simulink model "VFlexP"  (R2024a)
settings: Solver=ode23tb  StartTime=0.0  StopTime=3  FixedStep=1e-5
model workspace (MAT data in the model file):
  DCop_DCBUCK : object (value not decoded)
  Grid_CCVSC_idx = [2; 3; 4; 5; 6; 7; 8; 9; 10; 11; 12]
  Grid_CCVSCs = 1
  Grid_CCVSCs_buses = 1
  Grid_CCVSCs_toM = [0 1 0 0 0 0 0 0 0 0 0 0 ... (781 elements, 71x11)]
  Grid_C_Lines = [0 0]
  Grid_Cbuses = [0.00666666666667 0.00666666666667 0.00666666666667]
  Grid_DC : object (value not decoded)
  Grid_DCop_DCBUCK : object (value not decoded)
  Grid_DCop_DC_PES : object (value not decoded)
  Grid_DFIGs = 1
  Grid_DFIGs_buses = 1
  Grid_DGs : string (value not decoded)
  Grid_From_buses = [1 2]
  Grid_GFls = 1
  Grid_GFls_buses = 1
  Grid_GFr_idx = 1
  Grid_GFrs = 1
  Grid_GFrs_buses = 1
  Grid_GFrs_toM = [1; 0; 0]
  Grid_IG_idx = 2
  Grid_IGs = 1
  Grid_IGs_buses = 1
  Grid_IGs_toM = [0; 1]
  Grid_L_Lines = [0.05 0.05]
  Grid_L_Loads = 0
  Grid_Lines_fromM : object (value not decoded)
  Grid_Lines_toM : object (value not decoded)
  Grid_Load_buses = []
  Grid_Load_busesDC = []
  Grid_MSGs = 1
  Grid_MSGs_buses = 1
  Grid_Nbuses = 3
  Grid_PQ_gen = 3
  Grid_Ploads = []
  Grid_PloadsDC = []
  Grid_Ps_lf = -0.138475313333
  Grid_Qloads = []
  Grid_Qs_lf = 0.00594619333333
  Grid_R_Lines = [0.005 0.005]
  Grid_R_Loads = 0
  Grid_R_Loads_DC = 0
  Grid_Rcf = [150 150 150]
  Grid_SCs = 1
  Grid_SCs_buses = 1
  Grid_SG_idx = 1
  Grid_SGs = 1
  Grid_SGs_buses = 1
  Grid_SGs_toM = [1; 0]
  Grid_To_buses = [2 3]
  Grid_VCVSC_idx = [1; 2; 3; 4; 5; 6; 7; 8; 9; 10; 11; 12]
  Grid_VCVSCs = 1
  Grid_VCVSCs_buses = [1; 2; 3; 6; 8; 9; 12; 58; 59; 60; 63; 65]
  Grid_VCVSCs_toM = [1 0 0 0 0 0 0 0 0 0 0 0 ... (852 elements, 71x12)]
  Grid_VSM_idx = 2
  Grid_VSMs = 1
  Grid_VSMs_buses = 1
  Grid_VSMs_toM = [0; 1]
  Grid_admitt_matrix = [1.9801990198-19.801979198i  -1.9801980198+19.801980198i; -1.9801980198+19.801980198i  1.9801990198-19.801979198i]
  Grid_admitt_matrix_noloads = [1.9801990198-19.801979198i  -1.9801980198+19.801980198i; -1.9801980198+19.801980198i  1.9801990198-19.801979198i]
  Grid_bus = [1; 2; 3]
  Grid_busDC_complexity = 1
  Grid_busDC_complexity_PF = 2
  Grid_bus_complexity = [1 1 1]
  Grid_bus_complexity_PF = [1 1 1]
  Grid_buses_lf = 1
  Grid_conductance_matrix = 0.00666666666667
  Grid_conductance_matrix_noloads = 0.00666666666667
  Grid_fref : object (value not decoded)
  Grid_gen_static_params : mBase (value not decoded)
  Grid_iPs_lf = -7.22150378958
  Grid_iQs_lf = 168.17482109
  Grid_iadmitt_matrix = [250000.001075-249999.987531i  249999.998575-250000.012531i; 249999.998575-250000.012531i  250000.001075-249999.987531i]
  Grid_iadmitt_matrix_noloads = [250000.001075-249999.987531i  249999.998575-250000.012531i; 249999.998575-250000.012531i  250000.001075-249999.987531i]
  Grid_iconductance_matrix = 150
  Grid_iconductance_matrix_noloads = 150
  Grid_init_OK_bool = 1
  Grid_intconv_PF : object (value not decoded)
  Grid_lf_op : op_report (value not decoded)
  Grid_lineDC_complexity = []
  Grid_lineDC_complexity_PF = []
  Grid_line_complexity = [1 1]
  Grid_line_complexity_PF = [3 3]
  Grid_loadDC_complexity = []
  Grid_loadDC_complexity_PF = []
  Grid_load_complexity = []
  Grid_load_complexity_PF = []
  Grid_opDC_CCVSC : object (value not decoded)
  Grid_opDC_VSM : object (value not decoded)
  Grid_opGFr : object (value not decoded)
  Grid_opVCVSC : object (value not decoded)
  Grid_op_CCVSC : object (value not decoded)
  Grid_op_IG : object (value not decoded)
  Grid_op_SG : object (value not decoded)
  Grid_op_VSM : object (value not decoded)
  Grid_shift_lines = [0 0]
  Grid_tap_lines = [1 1]
  Grid_v_buses_mod = [1 1.0001218564 1]
  LinsysParamChangeStruct : Param1 (value not decoded)
  Lline = 0.01
  Rline = 1e-05
  linsys : object (value not decoded)
symbols that are objects in the model workspace (value not decoded): Grid_DCop_DC_PES, Grid_DCop_DCBUCK, Grid_op_CCVSC, Grid_op_IG, Grid_op_SG, Grid_op_VSM, Grid_opDC_CCVSC, Grid_opDC_VSM, Grid_opGFr, Grid_opVCVSC
undefined symbols (not defined in the file or in its folder): block_buses_DC, block_idx, CCVSC_idx, Cf, costs, costs2, DFIGs_nodes, DiscIntNeverNeededParam, entity, Fb, Fi, From_nodes, Grid_op_DFIG, Grid_op_DFIG_PQ, Grid_op_MSG, Grid_op_SC, Grid_op_VCVSC, Kic, Kiv, Kpc, Kpv, last_send, Lc, Lf, m, Matrix_flux_to_i, mD, mp, MSGs_buses, Nbuses_DC, nq, op_VCVSC, Psche, Rc, Rf, rkq1, rkq2, SCs_buses, SCs_nodes, sec_control_structure, set_DG_up, set_extra_satur, set_sending_cost, SGs_buses, SGs_nodes, Tf, To_nodes, VI_L, VI_R, WOF_Tf, xkq1, xkq2
libraries: simulink x447, eeGeneralControl x5
(part 2 of 30)

== system VFlexP/Grid/Dynamic/DCAC converters ==
  note: mdlWks = get_param(bdroot,'ModelWorkspace'); % Get the model workspace
      | block_name = get_param(gcb,'Name');
      | bvarname = get_param(get_param(get_param(get_param(...
      | gcb, 'Parent'), 'Parent'), 'Parent'), 'bvarname');
      | DC = mdlWks.getVariable([bvarname 'DC']);
      | try
      | block_DC_buses = DC.(block_name + "s_DC_buses");
      | block_buses = DC.(block_name + "s_buses");
      | block_DC_toM = DC.(block_name + "s_DC_toM");
      | block_toM = DC.(block_name + "s_toM");
      | dparams = DC.(block_name + "_dparams");
      | fref = mdlWks.getVariable([bvarname 'fref']);
      | block_fref = fref.(block_name);
      | catch ME
      | errordlg(ME.message)
      | end
  vac : Inport
  vdc : Inport  Port=2
  DC_CCVSC : Subsystem  Commented=on  mask(CCVSC){Pmax=0, Qmax=0, fb=50, dynamic_CC=Dynamic, Tint=0.1, Kint=1, Bint=1, dynamic_PLL=Dynamic, kpi=1, kii=10, Tf=0.01, alphapcoef=0, alphaqcoef=0, Prel=1, Qrel=1, Eref=1, kp=10, kq=10}
      mask prompts: Pmax "Active power limit (p.u.)"; Qmax "Reactive power limit (p.u.)"; fb "Base frequency (Hz)"; dynamic_CC "Dynamic behaviour"; dynamic_PLL "Dynamic behaviour"; Tf "LPF time constant (s)"; alphapcoef "P droop coefficient"; alphaqcoef "Q droop coefficient"; Prel "P/P_NmP"; Qrel "Q/Q_NnQ"; Eref "Nominal voltage of PCC"; kp "P gain"; kq "Q gain"
      mask help: Grid-following converter. CC is the current controller. Dynamic behavior includes the PI controller, decoupling and output inductance. Static behavior consists of setting the reference current directly in the output. PC is the power controller including the current reference calculation and low-pass filters for the power measurements.
      mask init:
      | mdlWks = get_param(bdroot,'ModelWorkspace'); % Get the model workspace
      | block_name = get_param(gcb,'Name');
      | bvarname = get_param(get_param(get_param(get_param(...
      |         gcb, 'Parent'), 'Parent'), 'Parent'), 'bvarname');
      | DC = mdlWks.getVariable([bvarname 'DC']);
      | try
      |     block_DC_buses = DC.(block_name + "s_DC_buses");
      |     block_buses = DC.(block_name + "s_buses");
      |     block_DC_toM = DC.(block_name + "s_DC_toM");
      |     block_toM = DC.(block_name + "s_toM");
      |     dparams = DC.(block_name + "_dparams");
      |     fref = mdlWks.getVariable([bvarname 'fref']);
      |     block_fref = fref.(block_name);
      | catch ME
      |     %errordlg(ME.message) 
      | end
      | 
      | 
      | block = gcb;
      | if Tf ~= 0
      |     iTf = 1/Tf;
      |     set_param([block '/PC/LPF_d'],'Commented','off')
      |     set_param([block '/PC/LPF_q'],'Commented','off')
      |     set_param([block '/LPF_d'],'Commented','off')
      |     set_param([block '/LPF_q'],'Commented','off')
      | else
      |     set_param([block '/PC/LPF_d'],'Commented','through')
      |     set_param([block '/PC/LPF_q'],'Commented','through')
      |     set_param([block '/LPF_d'],'Commented','through')
      |     set_param([block '/LPF_q'],'Commented','through')
      | end
      mask Help: web('Documentation/CCVSC.html')
      mask TypeOptions dynamic_CC: Dynamic | Static
      mask Callback dynamic_CC:
      | block = gcb;
      | dynamic = get_param(block, 'dynamic_CC');
      | param_vis = get_param(block,'MaskVisibilities');
      | block_params = string(fieldnames(get_param(block, 'DialogParameters')));
      | switch dynamic
      |     case 'Dynamic'
      |         set_param([gcb '/CC'], 'LabelModeActiveChoice', 'dynamic')
      |         param_vis(find(block_params == 'Tint'):find(block_params == 'Rf')) = cellstr("on");
      |     case 'Static'
      |         set_param([gcb '/CC'], 'LabelModeActiveChoice', 'static')
      |         param_vis(find(block_params == 'Tint'):find(block_params == 'Rf')) = cellstr("off");
      | end
      | set_param(block,'MaskVisibilities',param_vis)
      mask TypeOptions dynamic_PLL: Dynamic | Static
      mask Callback dynamic_PLL:
      | block = gcb;
      | dynamic = get_param(block, 'dynamic_PLL');
      | param_vis = get_param(block,'MaskVisibilities');
      | block_params = string(fieldnames(get_param(block, 'DialogParameters')));
      | switch dynamic
      |     case 'Dynamic'
      |         set_param([gcb '/PLL'], 'LabelModeActiveChoice', 'dynamic')
      |         param_vis(find(block_params == 'kpi'):find(block_params == 'kii')) = cellstr("on");
      |     case 'Static'
      |         set_param([gcb '/PLL'], 'LabelModeActiveChoice', 'static')
      |         param_vis(find(block_params == 'kpi'):find(block_params == 'kii')) = cellstr("off");
      | end
      | set_param(block,'MaskVisibilities',param_vis)
      mask DialogControl CC Prompt: CC
      mask DialogControl PLL Prompt: PLL
      mask DialogControl PC Prompt: PC
      mask DialogControl SC Prompt: SC
  DC_VCVSC : Subsystem  Commented=on  mask(VCVSC){Pmax=Inf, Qmax=Inf, fb=50, dynamic_VCC=Static, Lf=0.01, Rf=0.001, Rcf=1000000, Cfi=0.1, Kint=1, Tint=0.1, Bint=1, Kext=1, Bext=1, Text=0.1, Fi=1, Tf=0.01, mp=0.01, nq=0.01, VI_L=0.1, VI_R=0.01, WOF_Tf=0, cf=0.1, cv=0.1, L_out=0.1, R_out=0.01}
      mask prompts: Pmax "Active power limit (p.u.)"; Qmax "Reactive power limit (p.u.)"; fb "Base frequency (Hz)"; dynamic_VCC "Dynamic behavior"; Lf "Filter inductance (pu)"; Rf "Filter resistance (pu)"; Rcf "Parallel resistance to C (pu)"; Cfi "Filter capacitance (pu)"; Fi "Current feedfordward gain"; Tf "Low-pass filter time constant (s)"; mp "Droop coefficient mp (pu)"; nq "Droop coefficient nq (pu)"; VI_L "Inductance (pu)"; VI_R "Resistance (pu)"; WOF_Tf "WOF time constant (s)"; cf "Frequency SC gain"; cv "Voltage SC gain"; L_out "Output inductance (p.u.)"; R_out "Output resistance (p.u.)"
      mask help: Grid-forming converter. VCC are the voltage and current controllers. Dynamic behavior includes the PI controllers, decoupling, current feedfordward and LC output filter. Static behavior consists of setting the reference voltage directly in the output. PC is the power controller including the droop control and low-pass filters for the power measurements.
      mask init:
      | mdlWks = get_param(bdroot,'ModelWorkspace'); % Get the model workspace
      | block_name = get_param(gcb,'Name');
      | bvarname = get_param(get_param(get_param(get_param(...
      |         gcb, 'Parent'), 'Parent'), 'Parent'), 'bvarname');
      | DC = mdlWks.getVariable([bvarname 'DC']);
      | try
      |     block_DC_buses = DC.(block_name + "s_DC_buses");
      |     block_buses = DC.(block_name + "s_buses");
      |     block_DC_toM = DC.(block_name + "s_DC_toM");
      |     block_toM = DC.(block_name + "s_toM");
      |     dparams = DC.(block_name + "_dparams");
      | catch ME
      |     %errordlg(ME.message)
      | end
      mask Help: web('Documentation/VCVSC.html')
      mask TypeOptions dynamic_VCC: Dynamic with limitation | Dynamic | Static | Dynamic VC and static CC
      mask Callback dynamic_VCC:
      | block = gcb;
      | dynamic = get_param(block, 'dynamic_VCC');
      | param_vis = get_param(block,'MaskVisibilities');
      | block_params = string(fieldnames(get_param(block, 'DialogParameters')));
      | switch dynamic
      |     case 'Dynamic'
      |         param_vis(find(block_params == 'Lf'):find(block_params == 'Fi')) = cellstr("on");
      |         set_param([gcb '/VCC'], 'LabelModeActiveChoice', 'dynamic');
      |     case 'Dynamic with limitation'
      |         param_vis(find(block_params == 'Lf'):find(block_params == 'Fi')) = cellstr("on");
      |         set_param([gcb '/VCC'], 'LabelModeActiveChoice', 'dynamic_limiting');
      |     case 'Static'
      |         param_vis(find(block_params == 'Lf'):find(block_params == 'Fi')) = cellstr("off");
      |         set_param([gcb '/VCC'], 'LabelModeActiveChoice', 'static');
      |     case 'Dynamic VC and static CC'
      |         param_vis(find(block_params == 'Lf'):find(block_params == 'Fi')) = cellstr("on");
      |         param_vis(ismember(block_params, ["Lf","Rf","Kpc","Kic","Fi"])) = cellstr("off");
      |         set_param([gcb '/VCC'], 'LabelModeActiveChoice', 'dynamic_VC');
      | end
      | set_param(block,'MaskVisibilities',param_vis)
      mask TypeOptions Tf: PC/Tf
      mask TypeOptions mp: PC/mp
      mask TypeOptions nq: PC/nq
      mask TypeOptions VI_L: VI/L
      mask TypeOptions VI_R: VI/R
      mask TypeOptions WOF_Tf: VI/Tf
      mask DialogControl Container8 Prompt: Parameters
      mask DialogControl VCC Prompt: VCC
      mask DialogControl PC Prompt: PC
      mask DialogControl VI Prompt: VI
      mask DialogControl SC Prompt: SC
      mask DialogControl Container9 Prompt: Others
  DC_VSM : Subsystem  mask(VCVSC){Hv=Tf/(2*mp), Dv=0, Pmax=Inf, Qmax=Inf, fb=50, dynamic_VCC=Static, Lf=Lf, Rf=Rf, Rcf=1000000, Cfi=Cf, Kint=Kpc, Tint=Kpc/Kic, Bint=1, Kext=Kpv, Bext=1, Text=Kpv/Kiv, Fi=Fi, Rv=mp, nq=0, VI_L=VI_L, VI_R=VI_R, WOF_Tf=WOF_Tf, cf=0.1, cv=0.1, L_out=Lc, R_out=Rc}
      mask prompts: Hv "Inertia"; Dv "Damping"; Pmax "Active power limit (p.u.)"; Qmax "Reactive power limit (p.u.)"; fb "Base frequency (Hz)"; dynamic_VCC "Dynamic behavior"; Lf "Filter inductance (pu)"; Rf "Filter resistance (pu)"; Rcf "Parallel resistance to C (pu)"; Cfi "Filter capacitance (pu)"; Fi "Current feedfordward gain"; Rv "Droop Rv"; nq "Droop nq"; VI_L "Inductance (pu)"; VI_R "Resistance (pu)"; WOF_Tf "WOF time constant (s)"; cf "Frequency SC gain"; cv "Voltage SC gain"; L_out "Output inductance (p.u.)"; R_out "Output resistance (p.u.)"
      mask help: Grid-forming converter. VCC are the voltage and current controllers. Dynamic behavior includes the PI controllers, decoupling, current feedfordward and LC output filter. Static behavior consists of setting the reference voltage directly in the output. PC is the power controller including the droop control and low-pass filters for the power measurements.
      mask init: same as VFlexP/Grid/Dynamic/DCAC converters/DC_VCVSC
      mask Help: web('Documentation/VCVSC.html')
      mask TypeOptions dynamic_VCC: Dynamic with limitation | Dynamic | Static | Dynamic VC and static CC
      mask Callback dynamic_VCC:
      | block = gcb;
      | dynamic = get_param(block, 'dynamic_VCC');
      | param_vis = get_param(block,'MaskVisibilities');
      | block_params = string(fieldnames(get_param(block, 'DialogParameters')));
      | switch dynamic
      |     case 'Dynamic'
      |         param_vis(find(block_params == 'Lf'):find(block_params == 'Fi')) = cellstr("on");
      |         set_param([gcb '/VCC'], 'LabelModeActiveChoice', 'dynamic');
      |     case 'Dynamic with limitation'
      |         param_vis(find(block_params == 'Lf'):find(block_params == 'Fi')) = cellstr("on");
      |         set_param([gcb '/VCC'], 'LabelModeActiveChoice', 'dynamic_limiting');
      |     case 'Static'
      |         param_vis(find(block_params == 'Lf'):find(block_params == 'Fi')) = cellstr("off");
      |         set_param([gcb '/VCC'], 'LabelModeActiveChoice', 'static');
      |     case 'Dynamic VC and static CC'
      |         param_vis(find(block_params == 'Lf'):find(block_params == 'Fi')) = cellstr("on");
      |         param_vis(ismember(block_params, ["Lf","Rf","Kpc","Kic","Fi"])) = cellstr("off");
      |         set_param([gcb '/VCC'], 'LabelModeActiveChoice', 'dynamic_VC');
      | end
      | set_param(block,'MaskVisibilities',param_vis)
      mask TypeOptions VI_L: VI/L
      mask TypeOptions VI_R: VI/R
      mask TypeOptions WOF_Tf: VI/Tf
      mask DialogControl Container8 Prompt: Parameters
      mask DialogControl VCC Prompt: VCC
      mask DialogControl PC Prompt: PC
      mask DialogControl VI Prompt: VI
      mask DialogControl SC Prompt: SC
      mask DialogControl Container9 Prompt: Others
  Sum : Sum  Inputs=|+++
  Sum1 : Sum  Inputs=|+++
  iac : Outport
  idc : Outport  Port=2
  wires:
  [vac] -> DC_CCVSC/1(vac)
  [vac] -> DC_VCVSC/1(vac)
  vac/1 -> [vac]
  DC_VCVSC/1(iac) -> Sum/1
  Sum/1 -> iac/1
  DC_CCVSC/1(iac) -> Sum/2
  [vdc] -> DC_VCVSC/2(vdc)
  DC_VCVSC/2(idc) -> Sum1/1
  Sum1/1 -> idc/1
  DC_CCVSC/2(idc) -> Sum1/2
  [vdc] -> DC_CCVSC/2(vdc)
  vdc/1 -> [vdc]
  [vdc] -> DC_VSM/2(vdc)
  [vac] -> DC_VSM/1(vac)
  DC_VSM/2(idc) -> Sum1/3
  DC_VSM/1(iac) -> Sum/3

== system VFlexP/Grid/Dynamic/Generators ==
  note: Include the following mask initialisation code for each unit:
  note: mdlWks = get_param(bdroot,'ModelWorkspace'); % Get the model workspace
      | block_name = get_param(gcb,'Name');
      | try
      | bvarname = get_param(get_param(get_param(get_param(...
      | gcb, 'Parent'), 'Parent'), 'Parent'), 'bvarname');
      | block_buses = mdlWks.getVariable([bvarname block_name 's_buses']);
      | block_idx = mdlWks.getVariable([bvarname block_name '_idx']);
      | block_toM = mdlWks.getVariable([bvarname block_name 's_toM']);
      | fref = mdlWks.getVariable([bvarname 'fref']);
      | block_fref = fref.(block_name);
      | catch ME % block in initialisation
      | %errordlg(ME.message)
      | try
      | block_buses = 1:length(mdlWks.getVariable([block_name 's_buses']));
      | block_idx = mdlWks.getVariable([block_name '_idx']);
      | block_toM = mdlWks.getVariable([block_name 's_toM']);
      | block_fref = 1;
      | catch ME
      | %errordlg(ME.message)
      | end
      | end
  v : Inport
  ref : Inport  Port=2
  DFIG : Subsystem  Commented=on  mask(Doubly Fed Induction Generator){DFIGs_nodes=DFIGs_nodes, FBASE=50, D=0, H=3.3, Ls_pu=0.1178, Rs_pu=0.00734, Lm_pu=4.709, Rr_pu=0.01225, Lr_pu=0.15349, Ra_pu=0.1, La_pu=1, Cf_pu=0.0555, Ki_ia=7162, Kp_ia=6.5, Ki_ir=2117, Kp_ir=1.96, Ki_vc2=-562.5, Kp_vc2=-5.25, Ki_s=12000, Kp_s=1200, Kp_pll=2.33, Ki_pll=877}
      mask prompts: FBASE "Base frequency (Hz)"; D "Damping (pu)"; H "Inertia (s)"; Ls_pu "Stator inductances (pu)"; Rs_pu "Stator resistances (pu)"; Lm_pu "Mutual inductance (pu)"; Rr_pu "Rotor Resistance (pu)"; Lr_pu "Rotor Inductance"; Ra_pu "Filter Resistance (pu)"; La_pu "Filter Inductance (pu)"; Cf_pu "DC-Link Capacitance"; Ki_ia "GSC Ki"; Kp_ia "GSC Kp"; Ki_ir "RSC Ki"; Kp_ir "RSC Kp"; Ki_vc2 "DC Link Voltage Control Ki"; Kp_vc2 "DC Link Voltage Control Kp"; Ki_s "Slip Control Ki"; Kp_s "Slip Control Kp"; Kp_pll "PLL Kp"; Ki_pll "PLL Ki"
      mask help: Doubly Fed Induction Generator modelled in d-q reference frame.
      mask init:
      | mdlWks = get_param(bdroot,'ModelWorkspace'); % Get the model workspace
      | block_name = get_param(gcb,'Name');
      | try
      |     bvarname = get_param(get_param(get_param(get_param(...
      |         gcb, 'Parent'), 'Parent'), 'Parent'), 'bvarname');
      |     block_buses = mdlWks.getVariable([bvarname block_name 's_buses']);
      | 	block_idx = mdlWks.getVariable([bvarname block_name '_idx']);
      | catch % block in initialisation
      |     try
      |         block_buses = 1:length(mdlWks.getVariable([block_name 's_buses']));
      | 	    block_idx = mdlWks.getVariable([block_name '_idx']);
      |     catch ME
      |         %errordlg(ME.message)
      |     end
      | end
      | 
      | 
      |     n = length(block_buses);
      |     Lbiginv = zeros(6*n,6*n); % La grande con las inversas en diagonal
      |     if length(Ls_pu) == 1
      |         Ls_pu = Ls_pu*ones(1, n);
      |     end
      |     if length(Lr_pu) == 1
      |         Lr_pu = Lr_pu*ones(1, n);
      |     end
      |     if length(Lm_pu) == 1
      |         Lm_pu = Lm_pu*ones(1, n);
      |     end
      |     if length(La_pu) == 1
      |         La_pu = La_pu*ones(1, n);
      |     end
      |     Lss_pu =  Ls_pu + Lm_pu;
      |     Lrr_pu = Lr_pu + Lm_pu;
      |     
      |     for i=1:n
      |         j = 6*(i-1)+1;
      |         L = [Lss_pu(i) 0 Lm_pu(i) 0 0 0;...
      |         0 Lss_pu(i) 0 Lm_pu(i) 0 0;...
      |         Lm_pu(i) 0 Lrr_pu(i) 0 0 0;...
      |         0 Lm_pu(i) 0 Lrr_pu(i) 0 0;...
      |         0 0 0 0 La_pu(i) 0;...
      |         0 0 0 0 0 La_pu(i)];
      |         Lbiginv(j:j+5, j:j+5) = inv(L);
      |     end
      | %     sigma = Lrr_pu-(Lm_pu^2)/Lss_pu;
      |     sigma =  1-Lm_pu.^2./(Lss_pu.*Lrr_pu);
      |     omega_base = FBASE*2*pi;
      mask Help: web([extractBefore(get_param(bdroot, 'filename'),gcs) 'Documentation/SM.html'])
      mask DialogControl Params Prompt: Parameters
      mask DialogControl Container10 Prompt: PI Parameters
      mask DialogControl Params_copy Prompt: Parameters
  GFl : Subsystem  Commented=on  mask(GFl){Pmax=0, Qmax=0, fb=50, dynamic_CC=Static, Tint=0.1, Kint=1, Bint=1, Lf=0.01, Rf=0.001, dynamic_PLL=Dynamic, kpi=1, kii=10, Tf=0, alphapcoef=0, alphaqcoef=0, Prel=1, Qrel=1, Eref=1}
      mask prompts: Pmax "Active power limit (p.u.)"; Qmax "Reactive power limit (p.u.)"; fb "Base frequency (Hz)"; dynamic_CC "Dynamic behaviour"; Lf "Filter inductance"; Rf "Filter resistance"; dynamic_PLL "Dynamic behaviour"; Tf "LPF time constant (s)"; alphapcoef "P droop coefficient"; alphaqcoef "Q droop coefficient"; Prel "P/P_NmP"; Qrel "Q/Q_NnQ"; Eref "Nominal voltage of PCC"
      mask help: Grid-following converter. CC is the current controller. Dynamic behavior includes the PI controller, decoupling and output inductance. Static behavior consists of setting the reference current directly in the output. PC is the power controller including the current reference calculation and low-pass filters for the power measurements.
      mask init:
      | mdlWks = get_param(bdroot,'ModelWorkspace'); % Get the model workspace
      | block_name = get_param(gcb,'Name');
      | try
      |     bvarname = get_param(get_param(get_param(get_param(...
      |         gcb, 'Parent'), 'Parent'), 'Parent'), 'bvarname');
      |     block_buses = mdlWks.getVariable([bvarname block_name 's_buses']);
      | 	block_idx = mdlWks.getVariable([bvarname block_name '_idx']);
      |     block_toM = mdlWks.getVariable([bvarname block_name 's_toM']);
      |     fref = mdlWks.getVariable([bvarname 'fref']);
      |     block_fref = fref.(block_name);
      | catch ME % block in initialisation
      |     %errordlg(ME.message)
      |     try
      |         block_buses = 1:length(mdlWks.getVariable([block_name 's_buses']));
      | 	    block_idx = mdlWks.getVariable([block_name '_idx']);
      |         block_toM = mdlWks.getVariable([block_name 's_toM']);
      |         block_fref = 1;
      |     catch ME
      |         %errordlg(ME.message)
      |     end
      | end
      | 
      | 
      | 
      | block = gcb;
      | if Tf ~= 0
      |     iTf = 1/Tf;
      |     set_param([block '/PC/LPF_d'],'Commented','off')
      |     set_param([block '/PC/LPF_q'],'Commented','off')
      |     set_param([block '/LPF_d'],'Commented','off')
      |     set_param([block '/LPF_q'],'Commented','off')
      | else
      |     set_param([block '/PC/LPF_d'],'Commented','through')
      |     set_param([block '/PC/LPF_q'],'Commented','through')
      |     set_param([block '/LPF_d'],'Commented','through')
      |     set_param([block '/LPF_q'],'Commented','through')
      | end
      mask Help: web('doc_GFl.html')
      mask TypeOptions dynamic_CC: Dynamic | Static
      mask Callback dynamic_CC:
      | block = gcb;
      | dynamic = get_param(block, 'dynamic_CC');
      | param_vis = get_param(block,'MaskVisibilities');
      | block_params = string(fieldnames(get_param(block, 'DialogParameters')));
      | switch dynamic
      |     case 'Dynamic'
      |         set_param([gcb '/CC'], 'LabelModeActiveChoice', 'dynamic')
      |         param_vis(find(block_params == 'Tint'):find(block_params == 'Rf')) = cellstr("on");
      |     case 'Static'
      |         set_param([gcb '/CC'], 'LabelModeActiveChoice', 'static')
      |         param_vis(find(block_params == 'Tint'):find(block_params == 'Rf')) = cellstr("off");
      | end
      | set_param(block,'MaskVisibilities',param_vis)
      mask TypeOptions dynamic_PLL: Dynamic | Static
      mask Callback dynamic_PLL:
      | block = gcb;
      | dynamic = get_param(block, 'dynamic_PLL');
      | param_vis = get_param(block,'MaskVisibilities');
      | block_params = string(fieldnames(get_param(block, 'DialogParameters')));
      | switch dynamic
      |     case 'Dynamic'
      |         set_param([gcb '/PLL'], 'LabelModeActiveChoice', 'dynamic')
      |         param_vis(find(block_params == 'kpi'):find(block_params == 'kii')) = cellstr("on");
      |     case 'Static'
      |         set_param([gcb '/PLL'], 'LabelModeActiveChoice', 'static')
      |         param_vis(find(block_params == 'kpi'):find(block_params == 'kii')) = cellstr("off");
      | end
      | set_param(block,'MaskVisibilities',param_vis)
      mask DialogControl CC Prompt: CC
      mask DialogControl PLL Prompt: PLL
      mask DialogControl PC Prompt: PC
  GFr : Subsystem  mask(GFr){Pmax=Inf, Qmax=Inf, fb=50, dynamic_VCC=Static, Lf=0.1, Rf=0.01, Rcf=1000000, Cfi=0.1, Kint=1, Tint=0.1, Bint=1, Kext=0.1, Bext=1, Text=0.1, Fi=1, Tf=Tf, mp=mp, mD=mD, nq=0.001, VI_L=0, VI_R=0, WOF_Tf=0, L_out=Lc, R_out=Rc}
      mask prompts: Pmax "Active power limit (p.u.)"; Qmax "Reactive power limit (p.u.)"; fb "Base frequency (Hz)"; dynamic_VCC "Dynamic behavior"; Lf "Filter inductance (pu)"; Rf "Filter resistance (pu)"; Rcf "Parallel resistance to C (pu)"; Cfi "Filter capacitance (pu)"; Fi "Current feedfordward gain"; Tf "Low-pass filter time constant (s)"; mp "Droop coefficient mp (pu)"; mD "Droop coefficient mD (pu)"; nq "Droop coefficient nq (pu)"; VI_L "Inductance (pu)"; VI_R "Resistance (pu)"; WOF_Tf "WOF time constant (s)"; L_out "Output inductance (p.u.)"; R_out "Output resistance (p.u.)"
      mask help: Grid-forming converter. VCC are the voltage and current controllers. Dynamic behavior includes the PI controllers, decoupling, current feedfordward and LC output filter. Static behavior consists of setting the reference voltage directly in the output. PC is the power controller including the droop control and low-pass filters for the power measurements.
      mask init:
      | mdlWks = get_param(bdroot,'ModelWorkspace'); % Get the model workspace
      | block_name = get_param(gcb,'Name');
      | try
      |     bvarname = get_param(get_param(get_param(get_param(...
      |         gcb, 'Parent'), 'Parent'), 'Parent'), 'bvarname');
      |     block_buses = mdlWks.getVariable([bvarname block_name 's_buses']);
      | 	block_idx = mdlWks.getVariable([bvarname block_name '_idx']);
      |     block_toM = mdlWks.getVariable([bvarname block_name 's_toM']);
      |     fref = mdlWks.getVariable([bvarname 'fref']);
      |     block_fref = fref.(block_name);
      | catch ME % block in initialisation
      |     %errordlg(ME.message)
      |     try
      |         block_buses = 1:length(mdlWks.getVariable([block_name 's_buses']));
      | 	    block_idx = mdlWks.getVariable([block_name '_idx']);
      |         block_toM = mdlWks.getVariable([block_name 's_toM']);
      |         block_fref = 1;
      |     catch ME
      |         %errordlg(ME.message)
      |     end
      | end
      mask Help: web('doc_GFr.html')
      mask TypeOptions dynamic_VCC: Dynamic with limitation | Dynamic | Static | Dynamic VC and static CC
      mask Callback dynamic_VCC:
      | block = gcb;
      | dynamic = get_param(block, 'dynamic_VCC');
      | param_vis = get_param(block,'MaskVisibilities');
      | block_params = string(fieldnames(get_param(block, 'DialogParameters')));
      | switch dynamic
      |     case 'Dynamic'
      |         param_vis(find(block_params == 'Lf'):find(block_params == 'Fi')) = cellstr("on");
      |         set_param([gcb '/VCC'], 'LabelModeActiveChoice', 'dynamic');
      |     case 'Dynamic with limitation'
      |         param_vis(find(block_params == 'Lf'):find(block_params == 'Fi')) = cellstr("on");
      |         set_param([gcb '/VCC'], 'LabelModeActiveChoice', 'dynamic_limiting');
      |     case 'Static'
      |         param_vis(find(block_params == 'Lf'):find(block_params == 'Fi')) = cellstr("off");
      |         set_param([gcb '/VCC'], 'LabelModeActiveChoice', 'static');
      |     case 'Dynamic VC and static CC'
      |         param_vis(find(block_params == 'Lf'):find(block_params == 'Fi')) = cellstr("on");
      |         param_vis(ismember(block_params, ["Lf","Rf","Kpc","Kic","Fi"])) = cellstr("off");
      |         set_param([gcb '/VCC'], 'LabelModeActiveChoice', 'dynamic_VC');
      | end
      | set_param(block,'MaskVisibilities',param_vis)
      mask TypeOptions Tf: PC/Tf
      mask TypeOptions mp: PC/mp
      mask TypeOptions nq: PC/nq
      mask TypeOptions VI_L: VI/L
      mask TypeOptions VI_R: VI/R
      mask TypeOptions WOF_Tf: VI/Tf
      mask DialogControl Container8 Prompt: Parameters
      mask DialogControl VCC Prompt: VCC
      mask DialogControl PC Prompt: PC
      mask DialogControl VI Prompt: VI
      mask DialogControl Container9 Prompt: Others
  IG : Subsystem  Commented=on  mask{L_out_pu=0.1, R_out_pu=0.01}
      mask init: same as VFlexP/Grid/Dynamic/Generators/GFr
  MSG : Subsystem  Commented=on  mask(Doubly Fed Induction Generator){DFIGs_nodes=DFIGs_nodes, FBASE=50, D=0, H=7, Lssd_pu=1, Lssq_pu=0.6, Lmd_pu=0.9, Lmq_pu=0.5, Rs_pu=0.02, Lfd_pu=0.1, Rfd_pu=0.02, Rkd1_pu=10e6, Lkd1_pu=10e6, Rkd2_pu=10e6, Lkd2_pu=10e6, Rkq1_pu=10e6, Lkq1_pu=10e6, Rkq2_pu=10e6, Lkq2_pu=10e6, Rkq3_pu=10e6, Lkq3_pu=10e6, Ra_pu=0.008, La_pu=0.08, Cf_pu=0.0555, Ki_ia=0.1592, Kp_ia=9.1268e-04, Kid_m=1.9894, Kpd_m=0.0914, Kiq_m=1.1937, Kpq_m=0.0468, Ki_vc2=-0.1734, Kp_vc2=-0.0971, KPomegar=49, KIomegar=87.5, Kp_pll=9.1268e-05, Ki_pll=0.01592, T_e=1.15, T_1=12, T_2=1, T_A=0.01, K_A=200}
      mask prompts: FBASE "Base frequency (Hz)"; D "Damping (pu)"; H "Inertia (s)"; Lssd_pu "d-axis stator inductance (pu)"; Lssq_pu "q-axis stator inductance (pu)"; Lmd_pu "d-axis mutual inductance (pu)"; Lmq_pu "q-axis mutual inductance (pu)"; Rs_pu "Stator resistance (pu)"; Lfd_pu "Excitation indutance (pu)"; Rfd_pu "Excitation resistance (pu)"; Rkd1_pu "d-axis damper resistance 1 (pu)"; Lkd1_pu "d-axis damper inductance 1 (pu)"; Rkd2_pu "d-axis damper resistance 2 (pu)"; Lkd2_pu "d-axis damper inductance 2 (pu)"; Rkq1_pu "q-axis damper resistance 1(pu)"; Lkq1_pu "d-axis damper resistance 1 (pu)"; Rkq2_pu "d-axis damper resistance 2 (pu)"; Lkq2_pu "d-axis damper inductance 2 (pu)"; Rkq3_pu "d-axis damper resistance 3 (pu)"; Lkq3_pu "d-axis damper inductance 3 (pu)"; Ra_pu "Filter Resistance (pu)"; La_pu "Filter Inductance (pu)"; Cf_pu "DC-Link Capacitance"; Ki_ia "Grid side Converter Ki"; Kp_ia "Grid side Converter Kp"; Kid_m "d-axis Machine side Converter  Ki"; Kpd_m "d-axis Machine side Converter Kp"; Kiq_m "q-axis Machine side Converter  Ki"; Kpq_m "q-axis Machine side Converter Kp"; Ki_vc2 "DC Link Voltage Control Ki"; Kp_vc2 "DC Link Voltage Control Kp"; KPomegar "Speed control KP"; KIomegar "Speed control KI"; Kp_pll "PLL Kp"; Ki_pll "PLL Ki"
      mask help: Doubly Fed Induction Generator modelled in d-q reference frame.
      mask init:
      | mdlWks = get_param(bdroot,'ModelWorkspace'); % Get the model workspace
      | block_name = get_param(gcb,'Name');
      | try
      |     bvarname = get_param(get_param(get_param(get_param(...
      |         gcb, 'Parent'), 'Parent'), 'Parent'), 'bvarname');
      |     block_buses = mdlWks.getVariable([bvarname block_name 's_buses']);
      | 	block_idx = mdlWks.getVariable([bvarname block_name '_idx']);
      |     block_toM = mdlWks.getVariable([bvarname block_name 's_toM']);
      |     fref = mdlWks.getVariable([bvarname 'fref']);
      |     block_fref = fref.(block_name);
      | catch ME % block in initialisation
      |     %errordlg(ME.message)
      |     try
      |         block_buses = 1:length(mdlWks.getVariable([block_name 's_buses']));
      | 	    block_idx = mdlWks.getVariable([block_name '_idx']);
      |         block_toM = mdlWks.getVariable([block_name 's_toM']);
      |         block_fref = 1;
      |     catch ME
      |         %errordlg(ME.message)
      |     end
      | end
      |     
      | 
      | 
      | Lbiginv = zeros(6*length(block_buses),6*length(block_buses)); % La grande con las inversas en diagonal
      | for i=1:length(block_buses)
      |     j = 6*(i-1)+1;
      | %     L = [Lssd_pu(i)+Lmd_pu(i) 0 0 Lmd_pu(i) 0 0;...
      | %     0 Lssq_pu(i)+Lmq_pu(i) 0 0 0 0;...
      | %     0 0 Lssd_pu(i)-Lmd_pu(i) 0 0 0;...
      | %     Lmd_pu(i) 0 0 Lfd_pu(i)+Lmd_pu(i) 0 0;...
      | %     0 0 0 0 La_pu(i) 0;...
      | %     0 0 0 0 0 La_pu(i)];
      | 
      | Ldq0 = [Lssd_pu(i), 0 0; 0, Lssq_pu(i), 0; 0, 0, Lssd_pu(i)-Lmd_pu(i)]; 
      | Ladq0 = [Lmd_pu(i), 0, 0; 0, 0, 0; zeros(1, 3)];
      | Lk = [Lmd_pu(i) 0 0; zeros(1,3); zeros(1,3)] +...
      |     diag([Lfd_pu(i), La_pu(i), La_pu(i)]);
      | 
      | L = [Ldq0, Ladq0; Ladq0', Lk];
      |     Lbiginv(j:(j+5), j:(j+5)) = inv(L);
      | end
      | omega_base = FBASE*2*pi;
      mask Help: web([extractBefore(get_param(bdroot, 'filename'),gcs) 'Documentation/SM.html'])
      mask DialogControl Params Prompt: Parameters
      mask DialogControl Container10 Prompt: PI Parameters
      mask DialogControl Params_copy Prompt: Parameters
      mask DialogControl ContainerAVR Prompt: AVR Parameters
      mask DialogControl Params_AVR Prompt: Parameters
  SC : Subsystem  Commented=on  mask(Synchronous machine){SCs_nodes=SCs_nodes, FBASE=50, D=0, H=8, Psimag_pu=0.8, Lssd_pu=1.6, Lssq_pu=0.66, Rs_pu=0.0018, Lmd_pu=1.5, Lmq_pu=0.56, Rfd_pu=0.00052277, Lfd_pu=0.14234, Rkd1_pu=0.0168, Lkd1_pu=0.08125, Rkd2_pu=10e6, Lkd2_pu=10e6, Rkq1_pu=rkq1, Lkq1_pu=xkq1, Rkq2_pu=rkq2, Lkq2_pu=xkq2, Rkq3_pu=10e6, Lkq3_pu=10e6, T_e=1.15, T_1=12, T_2=1, T_A=0.01, K_A=200, R_p=0.05, T_W=2, R_t=0.43, T_g=0.5, T_R=9, Q=0, P=0, theta=0.9691426941, v=1}
      mask prompts: FBASE "Base frequency (Hz)"; D "Damping (pu)"; H "Inertia (s)"; Psimag_pu "Permanent flux (pu)"; Lssd_pu "Stator inductances (pu) Ld"; Lssq_pu "Stator inductances (pu) Lq"; Rs_pu "Stator resistances (pu)"; Lmd_pu "d-axis mutual inductance (pu)"; Lmq_pu "q-axis mutual inductance (pu)"; Rfd_pu "Excitation resistance (pu)"; Lfd_pu "Excitation inductance (pu)"; Rkd1_pu "d-axis damper resistance 1 (pu)"; Lkd1_pu "d-axis damper inductance 1 (pu)"; Rkd2_pu "d-axis damper resistance 2 (pu)"; Lkd2_pu "d-axis damper inductance 2 (pu)"; Rkq1_pu "q-axis damper resistance 1 (pu)"; Lkq1_pu "q-axis damper inductance 1 (pu)"; Rkq2_pu "q-axis damper resistance 2 (pu)"; Lkq2_pu "q-axis damper inductance 2 (pu)"; Rkq3_pu "q-axis damper resistance 3 (pu)"; Lkq3_pu "q-axis damper inductance 3 (pu)"; Q "Reactive power (pu)"; P "Active power (pu)"; theta "Voltage angle (pu)"; v "Voltage magnitude (pu)"
      mask help: Synchronous machine modelled in d-q reference frame.
      mask init:
      | mdlWks = get_param(bdroot,'ModelWorkspace'); % Get the model workspace
      | block_name = get_param(gcb,'Name');
      | try
      |     bvarname = get_param(get_param(get_param(get_param(...
      |         gcb, 'Parent'), 'Parent'), 'Parent'), 'bvarname');
      |     block_buses = mdlWks.getVariable([bvarname block_name 's_buses']);
      | 	block_idx = mdlWks.getVariable([bvarname block_name '_idx']);
      | catch % block in initialisation
      |     try
      |         block_buses = 1:length(mdlWks.getVariable([block_name 's_buses']));
      | 	    block_idx = mdlWks.getVariable([block_name '_idx']);
      |     catch ME
      |         %errordlg(ME.message)
      |     end
      | end
      | 
      |     
      | 
      |     Lbiginv = zeros(9*length(block_buses),9*length(block_buses)); % La grande con las inversas en diagonal
      |     for i=1:length(block_buses)
      |         j = 9*(i-1)+1;
      |         Ldq0 = [Lssd_pu(i), 0 0; 0, Lssq_pu(i), 0; 0, 0, 0.1]; % El 0.08 es del síncrono del lab
      |         Ladq0 = [Lmd_pu(i), Lmd_pu(i), Lmd_pu(i), 0 0 0; 0, 0, 0, Lmq_pu(i), Lmq_pu(i), Lmq_pu(i); zeros(1, 6)];
      |         Lk = [Lmd_pu(i)*ones(3,3), zeros(3,3); zeros(3,3), Lmq_pu(i)*ones(3,3)] +...
      |             diag([Lfd_pu(i), Lkd1_pu(i), Lkd2_pu(i), Lkq1_pu(i), Lkq2_pu(i), Lkq3_pu(i)]);
      |         L = [-Ldq0, Ladq0; -Ladq0', Lk];
      |         Lbiginv(j:(j+8), j:(j+8)) = inv(L);
      |     end
      mask Help: web([extractBefore(get_param(bdroot, 'filename'),gcs) 'Documentation/SM.html'])
      mask DialogControl Params Prompt: Parameters
      mask DialogControl AVR Prompt: AVR
      mask DialogControl Gov Prompt: Speed governor
      mask DialogControl op Prompt: Operating point
  SG : Subsystem  Commented=on  mask(Synchronous machine){SGs_nodes=SGs_nodes, FBASE=50, D=0.01, H=3.5, Psimag_pu=0.8, Lssd_pu=1.36*0+0.05*1, Lssq_pu=0.69*0+0.05*1 + 1.36*0, Rs_pu=0.005*0+0.01*1, Lmd_pu=1.28*0 + 0.04*1, Lmq_pu=1.28*0 + 0.04*1, Rfd_pu=0.0095*0+0.01*1, Lfd_pu=0.063*0+0.01*1, Rkd1_pu=0, Lkd1_pu=0, Rkd2_pu=0, Lkd2_pu=0, Rkq1_pu=0, Lkq1_pu=0, Rkq2_pu=0, Lkq2_pu=0, Rkq3_pu=0, Lkq3_pu=0, T_e=1.15, T_1=12, T_2=1, T_A=0.01, K_A=200, R_p=0.05, T_W=2, R_t=0.43, T_g=0.5, T_R=9}
      mask prompts: FBASE "Base frequency (Hz)"; D "Damping (pu)"; H "Inertia (s)"; Psimag_pu "Permanent flux (pu)"; Lssd_pu "Stator inductances (pu) Ld"; Lssq_pu "Stator inductances (pu) Lq"; Rs_pu "Stator resistances (pu)"; Lmd_pu "d-axis mutual inductance (pu)"; Lmq_pu "q-axis mutual inductance (pu)"; Rfd_pu "Excitation resistance (pu)"; Lfd_pu "Excitation inductance (pu)"; Rkd1_pu "d-axis damper resistance 1 (pu)"; Lkd1_pu "d-axis damper inductance 1 (pu)"; Rkd2_pu "d-axis damper resistance 2 (pu)"; Lkd2_pu "d-axis damper inductance 2 (pu)"; Rkq1_pu "q-axis damper resistance 1 (pu)"; Lkq1_pu "q-axis damper inductance 1 (pu)"; Rkq2_pu "q-axis damper resistance 2 (pu)"; Lkq2_pu "q-axis damper inductance 2 (pu)"; Rkq3_pu "q-axis damper resistance 3 (pu)"; Lkq3_pu "q-axis damper inductance 3 (pu)"
      mask help: Synchronous machine modelled in d-q reference frame.
      mask init:
      | mdlWks = get_param(bdroot,'ModelWorkspace'); % Get the model workspace
      | block_name = get_param(gcb,'Name');
      | try
      |     bvarname = get_param(get_param(get_param(get_param(...
      |         gcb, 'Parent'), 'Parent'), 'Parent'), 'bvarname');
      |     block_buses = mdlWks.getVariable([bvarname block_name 's_buses']);
      | 	block_idx = mdlWks.getVariable([bvarname block_name '_idx']);
      |     block_toM = mdlWks.getVariable([bvarname block_name 's_toM']);
      |     fref = mdlWks.getVariable([bvarname 'fref']);
      |     block_fref = fref.(block_name);
      | catch ME % block in initialisation
      |     %errordlg(ME.message)
      |     try
      |         block_buses = 1:length(mdlWks.getVariable([block_name 's_buses']));
      | 	    block_idx = mdlWks.getVariable([block_name '_idx']);
      |         block_toM = mdlWks.getVariable([block_name 's_toM']);
      |         block_fref = 1;
      |     catch ME
      |         %errordlg(ME.message)
      |     end
      | end
      | 
      |     
      | 
      |     
      |     n = length(block_buses);
      |     Lbiginv = zeros(9*n,9*n); % La grande con las inversas en diagonal
      |     if length(Lssd_pu) == 1
      |         Lssd_pu = Lssd_pu*ones(1, n);
      |     end
      |     if length(Lssq_pu) == 1
      |         Lssq_pu = Lssq_pu*ones(1, n);
      |     end
      |     if length(Lmd_pu) == 1
      |         Lmd_pu = Lmd_pu*ones(1, n);
      |     end
      |     if length(Lmq_pu) == 1
      |         Lmq_pu = Lmq_pu*ones(1, n);
      |     end
      |     if length(Lfd_pu) == 1
      |         Lfd_pu = Lfd_pu*ones(1, n);
      |     end
      |     if length(Lssd_pu) == 1
      |         Lssd_pu = Lssd_pu*ones(1, n);
      |     end
      |     if length(Lkd1_pu) == 1
      |         Lkd1_pu = Lkd1_pu*ones(1, n);
      |     end
      |     if length(Lkd2_pu) == 1
      |         Lkd2_pu = Lkd2_pu*ones(1, n);
      |     end
      |     if length(Lkq1_pu) == 1
      |         Lkq1_pu = Lkq1_pu*ones(1, n);
      |     end
      |     if length(Lkq2_pu) == 1
      |         Lkq2_pu = Lkq2_pu*ones(1, n);
      |     end
      |     if length(Lkq3_pu) == 1
      |         Lkq3_pu = Lkq3_pu*ones(1, n);
      |     end
      |     for i=1:n
      |         j = 9*(i-1)+1;
      |         Ldq0 = [Lssd_pu(i), 0 0; 0, Lssq_pu(i), 0; 0, 0, 0.0001]; % El 0.08 es del síncrono del lab
      |         Ladq0 = [Lmd_pu(i), Lmd_pu(i), Lmd_pu(i), 0 0 0; 0, 0, 0, Lmq_pu(i), Lmq_pu(i), Lmq_pu(i); zeros(1, 6)];
      |         Lk = [Lmd_pu(i)*ones(3,3), zeros(3,3); zeros(3,3), Lmq_pu(i)*ones(3,3)] +...
      |             diag([Lfd_pu(i), Lkd1_pu(i), Lkd2_pu(i), Lkq1_pu(i), Lkq2_pu(i), Lkq3_pu(i)]);
      |         L = [-Ldq0, Ladq0; -Ladq0', Lk];
      |         Lbiginv(j:(j+8), j:(j+8)) = inv(L);
      |     end
      mask Help: web([extractBefore(get_param(bdroot, 'filename'),gcs) 'Documentation/SM.html'])
      mask DialogControl Params Prompt: Parameters
      mask DialogControl AVR Prompt: AVR
      mask DialogControl Gov Prompt: Speed governor
  Signal Specification : SignalSpecification  Dimensions=[6 length(buses_lf) ]
  Signal Specification1 : SignalSpecification  Dimensions=[3 Nbuses]
  Sum : Sum  Inputs=|++++++++
  Sum2 : Sum  Inputs=|++++++++
  VSM : Subsystem  Commented=on  mask(VSM){Pmax=Inf, Qmax=Inf, fb=50, dynamic_VCC=Dynamic, Lf=Lf, Rf=Rf, Rcf=1000000, Cfi=Cf, Kint=Kpc, Tint=Kpc/Kic, Bint=1, Kext=Kpv, Bext=1, Text=Kpv/Kiv, Fi=Fi, Rv=mp, Dv=0, Hv=Tf/(2*mp), VI_L=VI_L, VI_R=VI_R, WOF_Tf=WOF_Tf, L_out=Lc, R_out=Rc}
      mask prompts: Pmax "Active power limit (p.u.)"; Qmax "Reactive power limit (p.u.)"; fb "Base frequency (Hz)"; dynamic_VCC "Dynamic behavior"; Lf "Filter inductance (pu)"; Rf "Filter resistance (pu)"; Rcf "Parallel resistance to C (pu)"; Cfi "Filter capacitance (pu)"; Fi "Current feedfordward gain"; Rv "Droop Rv"; Dv "Damping coefficient"; Hv "Inertia constant (s)"; VI_L "Inductance (pu)"; VI_R "Resistance (pu)"; WOF_Tf "WOF time constant (s)"; L_out "Output inductance (p.u.)"; R_out "Output resistance (p.u.)"
      mask help: Grid-forming converter working with VSM control. VCC are the voltage and current controllers. Dynamic behavior includes the PI controllers, decoupling, current feedfordward and LC output filter. Static behavior consists of setting the reference voltage directly in the output.
      mask init:
      | mdlWks = get_param(bdroot,'ModelWorkspace'); % Get the model workspace
      | block_name = get_param(gcb,'Name');
      | try
      |     bvarname = get_param(get_param(get_param(get_param(...
      |         gcb, 'Parent'), 'Parent'), 'Parent'), 'bvarname');
      |     block_buses = mdlWks.getVariable([bvarname block_name 's_buses']);
      | 	block_idx = mdlWks.getVariable([bvarname block_name '_idx']);
      |     block_toM = mdlWks.getVariable([bvarname block_name 's_toM']);
      |     fref = mdlWks.getVariable([bvarname 'fref']);
      |     block_fref = fref.(block_name);
      | catch ME % block in initialisation
      |     try
      |         block_buses = 1:length(mdlWks.getVariable([block_name 's_buses']));
      | 	    block_idx = mdlWks.getVariable([block_name '_idx']);
      |         block_toM = mdlWks.getVariable([block_name 's_toM']);
      |         block_fref = 1;
      |     catch ME
      |         %errordlg(ME.message)
      |     end
      | end
      mask Help: web('Documentation/VSM.html')
      mask TypeOptions dynamic_VCC: Dynamic with limitation | Dynamic | Static | Dynamic VC and static CC
      mask Callback dynamic_VCC:
      | block = gcb;
      | dynamic = get_param(block, 'dynamic_VCC');
      | param_vis = get_param(block,'MaskVisibilities');
      | block_params = string(fieldnames(get_param(block, 'DialogParameters')));
      | switch dynamic
      |     case 'Dynamic'
      |         param_vis(find(block_params == 'Lf'):find(block_params == 'Fi')) = cellstr("on");
      |         set_param([gcb '/VCC'], 'LabelModeActiveChoice', 'dynamic');
      |     case 'Dynamic with limitation'
      |         param_vis(find(block_params == 'Lf'):find(block_params == 'Fi')) = cellstr("on");
      |         set_param([gcb '/VCC'], 'LabelModeActiveChoice', 'dynamic_limiting');
      |     case 'Static'
      |         param_vis(find(block_params == 'Lf'):find(block_params == 'Fi')) = cellstr("off");
      |         set_param([gcb '/VCC'], 'LabelModeActiveChoice', 'static');
      |     case 'Dynamic VC and static CC'
      |         param_vis(find(block_params == 'Lf'):find(block_params == 'Fi')) = cellstr("on");
      |         param_vis(ismember(block_params, ["Lf","Rf","Kpc","Kic","Fi"])) = cellstr("off");
      |         set_param([gcb '/VCC'], 'LabelModeActiveChoice', 'dynamic_VC');
      | end
      | set_param(block,'MaskVisibilities',param_vis)
      mask TypeOptions VI_L: VI/L
      mask TypeOptions VI_R: VI/R
      mask TypeOptions WOF_Tf: VI/Tf
      mask DialogControl Container8 Prompt: Parameters
      mask DialogControl VCC Prompt: VCC
      mask DialogControl PC Prompt: PC
      mask DialogControl VI Prompt: VI
      mask DialogControl Container9 Prompt: Others
  i : Outport
  elec : Outport  Port=2
  wires:
  Sum/1 -> Signal Specification1/1
  Sum2/1 -> Signal Specification/1
  Signal Specification/1 -> elec/1
  Signal Specification1/1 -> i/1
  v/1 -> [v]
  [v] -> GFr/2(v)
  ref/1 -> [ref]
  [ref] -> GFr/1(elec_in)
  [ref] -> GFl/1(elec_in)
  [v] -> GFl/2(v)
  [v] -> SG/2(v)
  [ref] -> SG/1(elec_in)
  [ref] -> IG/1(elec_in)
  [v] -> IG/2(v)
  [v] -> SC/2(v)
  [ref] -> SC/1(elec_in)
  [ref] -> DFIG/1(elec_in)
  [v] -> DFIG/2(v)
  GFr/1(elec_out) -> Sum2/1
  GFl/1(elec_out) -> Sum2/2
  SG/1(elec_out) -> Sum2/3
  IG/1(elec_out) -> Sum2/4
  SC/1(elec_out) -> Sum2/5
  DFIG/1(elec_out) -> Sum2/6
  GFr/2(i) -> Sum/1
  GFl/2(i) -> Sum/2
  SG/2(i) -> Sum/3
  IG/2(i) -> Sum/4
  SC/2(i) -> Sum/5
  DFIG/2(i) -> Sum/6
  [v] -> VSM/2(v)
  [ref] -> VSM/1(elec_in)
  VSM/2(i) -> Sum/7
  VSM/1(elec_out) -> Sum2/7
  [v] -> MSG/2(v)
  [ref] -> MSG/1(elec_in)
  MSG/2(i) -> Sum/8
  MSG/1(elec_out) -> Sum2/8

== system VFlexP/Grid/Dynamic/Generators_DC ==
  note: mdlWks = get_param(bdroot,'ModelWorkspace'); % Get the model workspace
      | block_name = get_param(gcb,'Name');
      | try
      | bvarname = get_param(get_param(get_param(get_param(...
      | gcb, 'Parent'), 'Parent'), 'Parent'), 'bvarname');
      | DC = mdlWks.getVariable([bvarname 'DC']);
      | block_buses = DC.([block_name 's_buses']);
      | block_Pg = DC.([block_name 's_Pg']);
      | block_toM = DC.([block_name 's_toM']);
      | catch ME % block in initialisation
      | %errordlg(ME.message)
      | try
      | block_buses = 1:length(DC.([block_name 's_buses']));
      | block_Pg = DC.([block_name 's_Pg']);
      | block_toM = DC.([block_name 's_toM']);
      | catch ME
      | %errordlg(ME.message)
      | end
      | end
  v : Inport
  ref : Inport  Port=2
  DCBUCK : Subsystem  Commented=on
      mask init:
      | mdlWks = get_param(bdroot,'ModelWorkspace'); % Get the model workspace
      |     block_name = get_param(gcb,'Name');
      |     try
      |         bvarname = get_param(get_param(get_param(get_param(...
      |             gcb, 'Parent'), 'Parent'), 'Parent'), 'bvarname');
      |         DC = mdlWks.getVariable([bvarname 'DC']);
      |         block_buses = DC.([block_name 's_buses']);
      | 	    block_Pg = DC.([block_name 's_Pg']);
      |         block_toM = DC.([block_name 's_toM']);
      |     catch ME % block in initialisation
      |         %errordlg(ME.message)
      |         DC = mdlWks.getVariable('DC');
      |         try
      |             block_buses = 1:length(DC.([block_name 's_buses']));
      | 	        block_Pg = DC.([block_name 's_Pg']);
      |             block_toM = 1;
      |         catch ME
      |             %errordlg(ME.message)
      |         end
      |     end
  DC_PES : Subsystem
      mask init: same as VFlexP/Grid/Dynamic/Generators_DC/DCBUCK
  Sum : Sum  Inputs=|++
  i : Outport
  wires:
  v/1 -> [v]
  ref/1 -> [ref]
  [v] -> DCBUCK/1(v)
  [ref] -> DCBUCK/2(ref)
  [ref] -> DC_PES/2(ref)
  [v] -> DC_PES/1(v)
  Sum/1 -> i/1
  DCBUCK/1(i) -> Sum/1
  DC_PES/1(i) -> Sum/2

== system VFlexP/Grid/Dynamic/Grid ==
  note: 1) Add Subsystem or Model blocks as valid variant choices.
      | 2) You cannot connect blocks at this level. At simulation, connectivity is automatically
      | determined, based on the active variant and port name matching.
  i_from_gen : Inport
  Dynamic : Subsystem  VariantControl=Dynamic
  Static : Subsystem  VariantControl=Static
  v_buses : Outport

== system VFlexP/Grid/Dynamic/Grid_DC ==
  note: 1) Add Subsystem or Model blocks as valid variant choices.
      | 2) You cannot connect blocks at this level. At simulation, connectivity is automatically
      | determined, based on the active variant and port name matching.
  i_from_gen_dc : Inport
  dynamic : Subsystem  VariantControl=Dynamic
  static : Subsystem  VariantControl=Static
  v_buses_dc : Outport

== system VFlexP/Grid/Dynamic/LPF ==
  In1 : Inport
  Gain : Gain  Gain=1e2
  I : Integrator  InitialCondition=1
  Sum4 : Sum  Inputs=|+-
  Out1 : Outport
  wires:
  Gain/1 -> I/1
  Sum4/1 -> Gain/1
  In1/1 -> Sum4/1
  I/1 -> Out1/1, Sum4/2

== system VFlexP/Grid/Dynamic/LPF1 ==
  In1 : Inport
  Gain : Gain  Gain=1e2
  I : Integrator  InitialCondition=Ps_lf
  Sum4 : Sum  Inputs=|+-
  Out1 : Outport
  wires:
  I/1 -> Sum4/2, Out1/1
  In1/1 -> Sum4/1
  Sum4/1 -> Gain/1
  Gain/1 -> I/1

== system VFlexP/Grid/Dynamic/LPF2 ==
  In1 : Inport
  Gain : Gain  Gain=1e2
  I : Integrator  InitialCondition=v_buses_mod(buses_lf)
  Sum4 : Sum  Inputs=|+-
  Out1 : Outport
  wires:
  Gain/1 -> I/1
  Sum4/1 -> Gain/1
  In1/1 -> Sum4/1
  I/1 -> Out1/1, Sum4/2
